simulink model "Camera"  (R2023b)
settings: Solver=VariableStepAuto  StartTime=0.0  StopTime=10.0  RelTol=1e-3
settings Model: Creator=user  LastModifiedBy=user

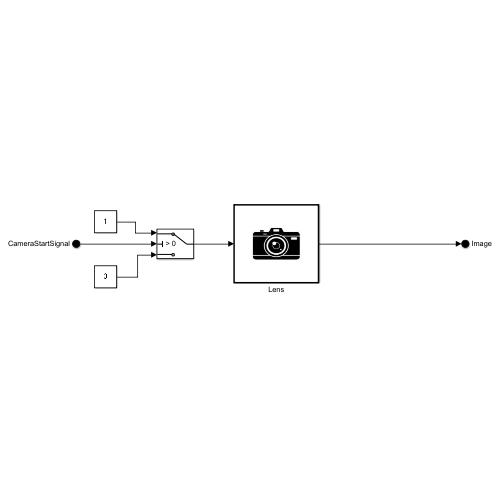
[thumbnail: Simulink's stored preview of the top-level diagram]
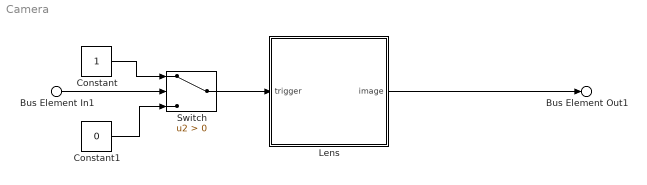
== system Camera ==
  Bus Element In1 : Inport  PortName=CameraStartSignal
  Constant : Constant
  Constant1 : Constant  Value=0
  Lens : MATLAB Function  TreatAsAtomicUnit=on
  Switch : Switch  Criteria=u2 > Threshold  SaturateOnIntegerOverflow=off  InputSameDT=off
  Bus Element Out1 : Outport  PortName=Image
  wires:
  Bus Element In1/1 -> Switch/2
  Constant/1 -> Switch/1
  Constant1/1 -> Switch/3
  Switch/1 -> Lens/1(trigger)
  Lens/1(image) -> Bus Element Out1/1

== matlab function Camera/Lens ==
  data: trigger input; image output
function image = fcn(trigger)
if trigger>0
    image = 255*rand(200, 200);
else
    image = zeros(200,200);
end
